simulink library "PID_library"  (R2020a)
settings: Solver=VariableStepAuto  StartTime=0.0  StopTime=10.0  RelTol=1e-3
undefined symbols (not defined in the file): kd, ki, kp, T, tau
settings Model: Creator=muril  LastModifiedBy=muril

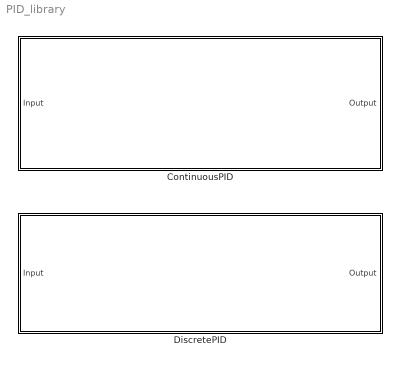
== system PID_library ==
  ContinuousPID : Subsystem
  DiscretePID : Subsystem

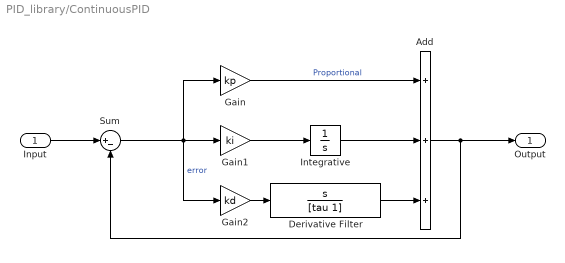
== system PID_library/ContinuousPID ==
  Input : Inport
  Add : Sum  Inputs=+++
  Derivative Filter : TransferFcn  Numerator=[1 0]  Denominator=[tau 1]  ContinuousStateAttributes='D'
  Gain : Gain  Gain=kp
  Gain1 : Gain  Gain=ki
  Gain2 : Gain  Gain=kd
  Integrative : Integrator  ContinuousStateAttributes='I'
  Sum : Sum  Inputs=|+-
  Output : Outport
  wires:
  Sum/1 -> Gain/1, Gain2/1, Gain1/1  "error"
  Derivative Filter/1 -> Add/3
  Gain2/1 -> Derivative Filter/1
  Input/1 -> Sum/1
  Add/1 -> Output/1, Sum/2
  Gain/1 -> Add/1  "Proportional"
  Gain1/1 -> Integrative/1
  Integrative/1 -> Add/2

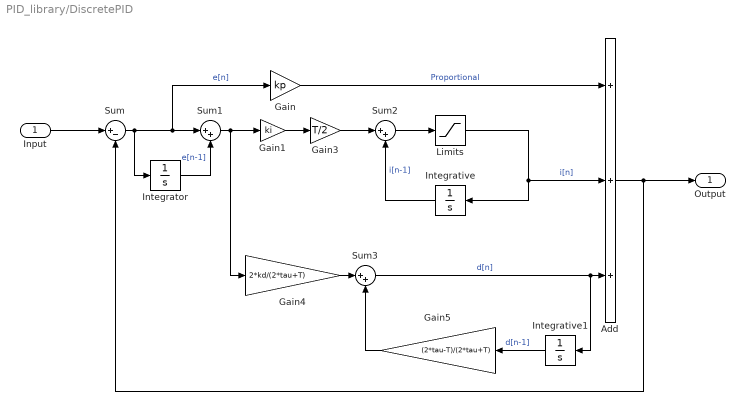
== system PID_library/DiscretePID ==
  Input : Inport
  Add : Sum  Inputs=+++
  Gain : Gain  Gain=kp
  Gain1 : Gain  Gain=ki
  Gain3 : Gain  Gain=T/2
  Gain4 : Gain  Gain=2*kd/(2*tau+T)
  Gain5 : Gain  Gain=(2*tau-T)/(2*tau+T)
  Integrative : Integrator  ContinuousStateAttributes='PrevI'
  Integrative1 : Integrator  ContinuousStateAttributes='PrevD'
  Integrator : Integrator  ContinuousStateAttributes='PrevE
  Limits : Saturate  LowerLimit=0.001
  Sum : Sum  Inputs=|+-
  Sum1 : Sum  Inputs=|++
  Sum2 : Sum  Inputs=|++
  Sum3 : Sum  Inputs=|++
  Output : Outport
  wires:
  Gain3/1 -> Sum2/1
  Sum1/1 -> Gain4/1, Gain1/1
  Add/1 -> Output/1, Sum/2
  Sum/1 -> Integrator/1, Sum1/1, Gain/1  "e[n]"
  Integrative1/1 -> Gain5/1  "d[n-1]"
  Integrator/1 -> Sum1/2  "e[n-1]"
  Gain5/1 -> Sum3/2
  Sum2/1 -> Limits/1
  Integrative/1 -> Sum2/2  "i[n-1]"
  Limits/1 -> Integrative/1, Add/2  "i[n]"
  Gain/1 -> Add/1  "Proportional"
  Input/1 -> Sum/1
  Gain1/1 -> Gain3/1
  Sum3/1 -> Integrative1/1, Add/3  "d[n]"
  Gain4/1 -> Sum3/1
